simulink model "Boat_model_thrust"  (Simulink 6.6)
settings: Solver=ode3  StartTime=0.0  StopTime=1000.0  FixedStep=1  RelTol=1e-3
libraries: simulink x2
settings Model: Creator=Administrator  LastModifiedBy=Administrator

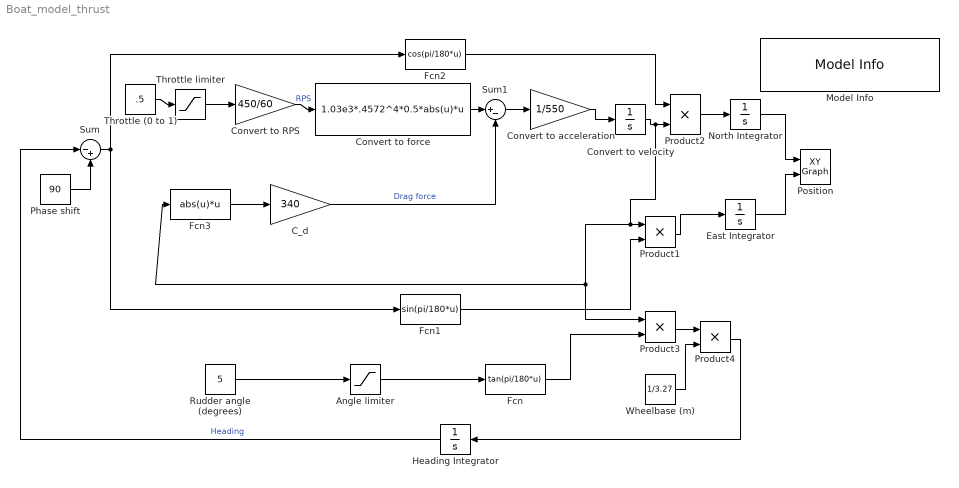
== system Boat_model_thrust ==
  Angle limiter : Saturate  UpperLimit=60  LowerLimit=-60
  C_d : Gain  Gain=340
  Convert to RPS : Gain  Gain=450/60
  Convert to acceleration : Gain  Gain=1/550
  Convert to force : Fcn  Expr=1.03e3*.4572^4*0.5*abs(u)*u
  Convert to velocity : Integrator
  East Integrator : Integrator
  Fcn : Fcn  Expr=tan(pi/180*u)
  Fcn1 : Fcn  Expr=sin(pi/180*u)
  Fcn2 : Fcn  Expr=cos(pi/180*u)
  Fcn3 : Fcn  Expr=abs(u)*u
  Heading Integrator : Integrator  Orientation=left
  Model Info : simulink/Model-Wide Utilities/Model Info  SystemSampleTime=-1  InitialBlockCM=None  BlockCM=None  Frame=on  DisplayStringWithTags=|  HorizontalTextAlignment=Center  LeftAlignmentValue=0.5  SourceBlockDiagram=Boat_model_thrust  TagMaxNumber=20
      | Kinematic model of the autoboat.
      | Version %<ModelVersion>
  North Integrator : Integrator
  Phase shift : Constant  Value=90
  Position : simulink/Sinks/XY Graph  SystemSampleTime=-1  xmin=-10000  xmax=10000  ymin=-10000  ymax=10000  st=-1
  Product{1..4} (4 alike) : Product  RndMeth=Zero
  Rudder angle (degrees) : Constant  Value=5
  Sum : Sum  Inputs=|-+
  Sum1 : Sum  Inputs=|+-
  Throttle (0 to 1) : Constant  Value=.5
  Throttle limiter : Saturate  UpperLimit=1  LowerLimit=0
  Wheelbase (m) : Constant  Value=1/3.27
  wires:
  Rudder angle (degrees)/1 -> Angle limiter/1
  North Integrator/1 -> Position/1
  Fcn2/1 -> Product2/1
  East Integrator/1 -> Position/2
  Fcn1/1 -> Product1/2
  Product2/1 -> North Integrator/1
  Fcn/1 -> Product3/2
  Wheelbase (m)/1 -> Product4/2
  Product3/1 -> Product4/1
  Sum/1 -> Fcn2/1, Fcn1/1
  Phase shift/1 -> Sum/2
  Product1/1 -> East Integrator/1
  Angle limiter/1 -> Fcn/1
  Product4/1 -> Heading Integrator/1
  Heading Integrator/1 -> Sum/1  "Heading"
  Throttle (0 to 1)/1 -> Throttle limiter/1
  Throttle limiter/1 -> Convert to RPS/1
  Convert to RPS/1 -> Convert to force/1  "RPS"
  Convert to velocity/1 -> Product2/2, Product1/1, Product3/1, Fcn3/1
  Fcn3/1 -> C_d/1
  C_d/1 -> Sum1/2  "Drag force"
  Convert to acceleration/1 -> Convert to velocity/1
  Sum1/1 -> Convert to acceleration/1
  Convert to force/1 -> Sum1/1
